simulink model "embedded"  (Simulink 7.3)
settings: Solver=FixedStepDiscrete  StartTime=0.0  StopTime=10.0  FixedStep=1  RelTol=1e-3
settings Model: Creator=hnine  LastModifiedBy=hnine
settings OptimizationCC: InitFltsAndDblsToZero=on
settings DebuggingCC: SaveWithParameterizedLinksMsg=none
settings GRTTargetCC: TargetFcnLib=ansi_tfl_tmw.mat

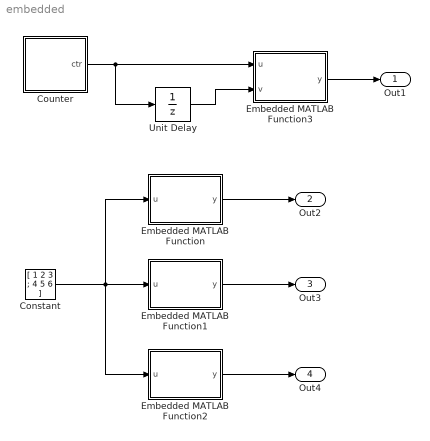
== system embedded ==
  Constant : Constant  Value=[ 1 2 3 ; 4 5 6 ]  VectorParams1D=off  OutDataType=sfix(16)  OutScaling=2^0
  Counter : Stateflow chart
  Embedded MATLAB Function : Stateflow chart
  Embedded MATLAB Function1 : Stateflow chart
  Embedded MATLAB Function2 : Stateflow chart
  Embedded MATLAB Function3 : Stateflow chart
  Unit Delay : UnitDelay
  Out1 : Outport  OutDataType=sfix(16)  OutScaling=2^0
  Out2 : Outport  Port=2  OutDataType=sfix(16)  OutScaling=2^0
  Out3 : Outport  Port=3  OutDataType=sfix(16)  OutScaling=2^0
  Out4 : Outport  Port=4  OutDataType=sfix(16)  OutScaling=2^0
  wires:
  Constant/1 -> Embedded MATLAB Function/1(u), Embedded MATLAB Function1/1(u), Embedded MATLAB Function2/1(u)
  Embedded MATLAB Function/1(y) -> Out2/1
  Embedded MATLAB Function1/1(y) -> Out3/1
  Embedded MATLAB Function2/1(y) -> Out4/1
  Counter/1(ctr) -> Embedded MATLAB Function3/1(u), Unit Delay/1
  Unit Delay/1 -> Embedded MATLAB Function3/2(v)
  Embedded MATLAB Function3/1(y) -> Out1/1

== matlab function Embedded MATLAB Function1 ==
  data: u input double; y output double
function y = fcn(u)
% This block supports an embeddable subset of the MATLAB language.
% See the help menu for details. 

y = u(2,:);

== matlab function Embedded MATLAB Function ==
  data: u input double; y output double
function y = fcn(u)
% This block supports an embeddable subset of the MATLAB language.
% See the help menu for details. 

y = u(1);

== matlab function Embedded MATLAB Function2 ==
  data: u input double; y output double
function y = fcn(u)
% This block supports an embeddable subset of the MATLAB language.
% See the help menu for details. 

y = u(:,3);

== stateflow chart Counter ==
  state s1
  (default) -> s1
  s1 -> s1 [order 1] : [ctr < 4] / ctr = ctr+1;
  s1 -> s1 [order 2] : [ctr >= 4] / ctr = 0;
  data: ctr output double =1

== matlab function Embedded MATLAB Function3 ==
  data: u input double; y output double; v input double
function y = fcn(u, v)
% This block supports an embeddable subset of the MATLAB language.
% See the help menu for details. 

y = u + v;
